simulink model "Q5"  (R2023a)
settings: Solver=VariableStepAuto  StartTime=0.0  StopTime=50  RelTol=1e-3
undefined symbols (not defined in the file): Aobs, B, L
libraries: simulink_extras x2
settings Model: Creator=anshu  LastModifiedBy=anshu

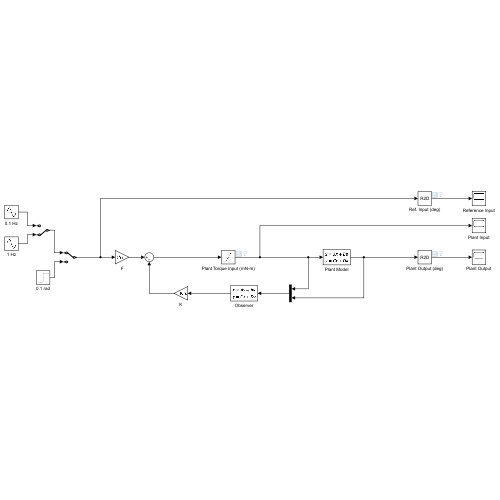
[thumbnail: Simulink's stored preview of the top-level diagram]
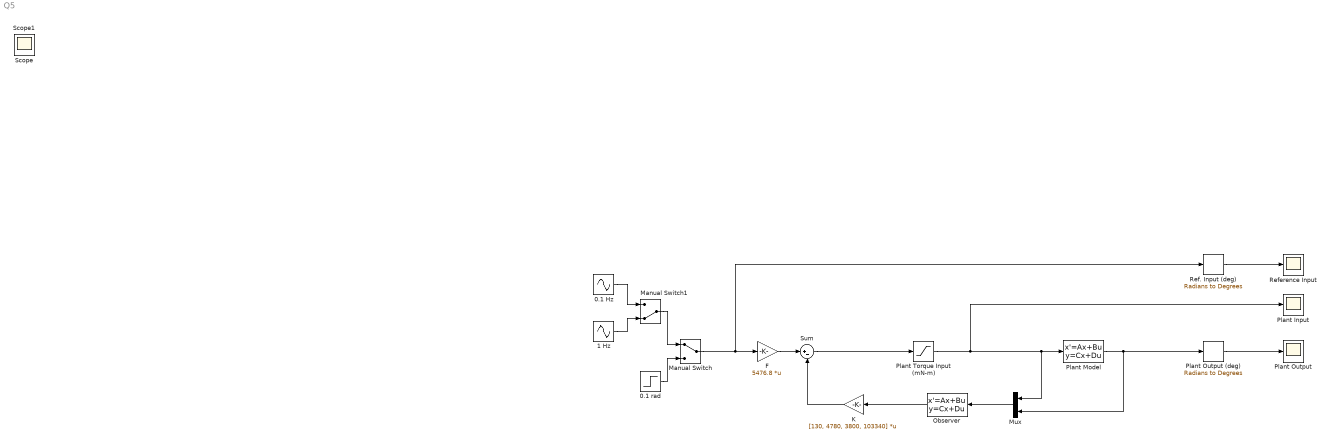
== system Q5 ==
  0.1 Hz : Sin  Amplitude=2.5  Frequency=0.628  SampleTime=0
  0.1 rad : Step  After=0.1  SampleTime=0
  1 Hz : Sin  Amplitude=0.3  Frequency=6.28  SampleTime=0
  F : Gain  Gain=5476.8  Multiplication=Matrix(K*u)
  K : Gain  Gain=[130, 4780, 3800, 103340]  Multiplication=Matrix(K*u)
  Manual Switch : ManualSwitch
  Manual Switch1 : ManualSwitch  CurrentSetting=0
  Mux : Mux  Inputs=2
  Observer : StateSpace  A=Aobs  B=[B, L]  C=eye(4)  D=zeros(4,2)  InitialCondition=0  ParameterTunability=Unconstrained
  Plant Input : Scope
  Plant Model : StateSpace  A=[-5.2954, -70.1022, -343.1258, 0; 1, 0, 0, 0; 0, 1, 0, 0; 0, 0, 1, 0]  B=[1; 0; 0; 0]  C=[0, 0.8913, 0.1603, 18.8679]  D=0  InitialCondition=0  ParameterTunability=Unconstrained
  Plant Output : Scope
  Plant Output (deg) : simulink_extras/Transformations/Radians to Degrees
  Plant Torque Input (mN-m) : Saturate  UpperLimit=67  LowerLimit=-67
  Ref. Input (deg) : simulink_extras/Transformations/Radians to Degrees
  Reference Input : Scope
  Sum : Sum  Inputs=|+-
  Scope : Scope
  Scope1 : Scope
  wires:
  Manual Switch/1 -> Ref. Input (deg)/1, F/1
  Manual Switch1/1 -> Manual Switch/1
  1 Hz/1 -> Manual Switch1/2
  Sum/1 -> Plant Torque Input (mN-m)/1
  Ref. Input (deg)/1 -> Reference Input/1
  0.1 rad/1 -> Manual Switch/2
  Plant Output (deg)/1 -> Plant Output/1
  K/1 -> Sum/2
  F/1 -> Sum/1
  0.1 Hz/1 -> Manual Switch1/1
  Plant Torque Input (mN-m)/1 -> Plant Model/1, Mux/1, Plant Input/1
  Observer/1 -> K/1
  Mux/1 -> Observer/1
  Plant Model/1 -> Plant Output (deg)/1, Mux/2
